simulink model "HPWnew"  (R2015a)
settings: Solver=ode45  StartTime=0.0  StopTime=10.0  RelTol=1e-3
undefined symbols (not defined in the file): c1, c2, c3, c4, c5, c6, Hydride, Metal, Nickel, PV1, PV2, PV3
libraries: powerlib x263, electricdrivelib x30, powerlib_meascontrol x15, powerlib_extras x7, re_lib x3, fuzblock x3, simulink x2
(part 4 of 8)

== system HPWnew/Wind Power System 60 KW x 25 = 1.5MW/Wind 60KW, 50HZ, 440V19 ==
  "Gen Speed " : Inport
  PA (deg) : Inport  Port=2
  Wind Speed (m/s) : Inport  Port=3
  Ground (output) : powerlib/Elements/Ground  LConnTagsString=a
  Load Flow Bus : powerlib/Measurements/Load Flow Bus  LConnTagsString=a  ID=B1  Vbase=762.1  Vref=1  Vangle=0  VLF=1  angleLF=-0.3472
      settings: AttributesFormatString=%<ID>\n%<Vbase>V\n%<VLF>pu\n%<angleLF>deg.
  Network 440Vrms LN - 10 MVA : powerlib/Electrical Sources/Three-Phase Source  Voltage=(762.1)*1  PhaseAngle=0  Frequency=60  InternalConnection=Yn  SpecifyImpedance=off  Resistance=762^2/10e6/10  Inductance=762^2/10e6/(2*pi*60)  ShortCircuitLevel=100e6  BaseVoltage=25e3  XRratio=7  BusType=swing  Pref=0  Qref=0  Qmin=-Inf  Qmax=Inf
  Scope : Scope  NumInputPorts=2
      settings: TimeRange=0.05586047612700701  YMin=-800~-200  YMax=800~200
  Synchronous Machine 762 V 111.9 kW : powerlib/Machines/Synchronous Machine SI Fundamental  PresetModel=05: 50Hz 400V 60kVA 1500RPM  MechanicalLoad=Mechanical power Pm  ShowDetailedParameters=on  RotorType=Salient-pole  Units=SI fundamental parameters  MeasurementBus=off  NominalParameters=[6e+04 400 50]  Stator=[0.101 0.0006791 0.01833 0.007979]  Field=[0.05664 0.001459]  Dampers2=[ 1 2 3 4 5 6 ]  Dampers1=[0.3901 0.002619 0.1534 0.0004483]  Mechanical=[0.5 0.05 2]  PolePairs=2  InitialConditions=[0 -111.483 53.977 53.977 53.977 -173.297 -293.297 -53.2967 17.8876]  SetSaturation=off  Saturation=[46.376,51.647,61.167,66.773,72.147,78.393,86.24,95.347,105.58;644,708.2,816.2,870.87,917.13,962.47,1012,1059.3,1104.5]  DisplayVfd=off  LoadFlowParameters=[1 -50000 0 0 0]  TsPowergui=0  TsBlock=-1  IterativeModel=Forward Euler  BusType=PV  Pref=-50000  Qref=0  Qmin=-Inf  Qmax=Inf  PLF=0  QLF=0
      settings: AttributesFormatString=\n
  Three-Phase Series RLC Load : powerlib/Elements/Three-Phase Series RLC Load  LConnTagsString=A|B|C  Configuration=Y (grounded)  NominalVoltage=440  NominalFrequency=50  ActivePower=10e3  InductivePower=0  CapacitivePower=0  Measurements=None  LoadType=constant Z
  Three-Phase V-I Measurement : powerlib/Measurements/Three-Phase V-I Measurement  VoltageMeasurement=phase-to-ground  SetLabelV=off  LabelV=Vabc  Vpu=off  VpuLL=off  CurrentMeasurement=yes  SetLabelI=off  LabelI=Iabc  Ipu=off  Pbase=100e6  Vbase=500e3  OutputType=Complex  PhasorSimulation=off  PSBequivalent=0
  Wind Turbine : Subsystem  AncestorBlock=re_lib/Wind Generation/Wind Turbine  DialogController=POWERSYS.PowerSysDialog  mask(Wind Turbine){Pnom=1.5e6, Pelec_base=1.5e6/0.9, wind_base=12, P_wind_base=0.73, speed_nom=1.2, pitch_angle=0, DisplayTurbChar=off, c1_c6=[0.51763          116          0.4            5           21     0.006795], cp_nom=0.48, lambda_nom=8.1}
      mask prompts: Pnom "Nominal mechanical output power (W):"; Pelec_base "Base power of the electrical generator (VA):"; wind_base "Base wind speed (m/s):"; P_wind_base "Maximum power at base wind speed (pu of nominal mechanical power):"; speed_nom "Base rotational speed (p.u. of base generator speed):"; pitch_angle "Pitch angle beta to display wind-turbine power characteristics (beta >=0)  (deg):"; DisplayTurbChar "Display wind turbine power characteristics"
      mask help:
      | This block implements a variable pitch wind turbine model. The performance coefficient Cp of the turbine is the mechanical output power of the turbine divided by wind power and a function of wind speed, rotational speed, and pitch angle (beta). Cp reaches its maximum value at zero beta. Select the wind-turbine power characteristics display to plot the turbine characteristics at the specified pitch angle.
      |
      | The first input is the generator speed in per unit of the generator base speed. For a synchronous or asynchronous generator, the base speed is the synchronous speed. For a permanent-magnet generator, the base speed is defined as the speed producing nominal voltage at  no load. The second input is the blade pitch angle (beta) in degrees. The third input is the wind speed in m/s.
      |
      | The output is the torque applied to the generator shaft in per unit of the generator ratings.
      |
      | The turbine inertia must be added to the generator inertia.
      mask init: same as HPWnew/Wind Power System 60 KW x 25 = 1.5MW/Wind 60KW, 50HZ, 440V1/Wind Turbine
      mask Help: helpview(psbhelp);
      mask Callback Pnom:
      | ParVisible={'on','on','on','on','on','on','on','off','off','off',};
      | set_param(gcb,'MaskVisibilities',ParVisible);
      | c1_c6=str2num(get_param(gcb,'c1_c6'));
      | c1=c1_c6(1);c2=c1_c6(2);c3=c1_c6(3);c4=c1_c6(4);c5=c1_c6(5);c6=c1_c6(6);
      mask Callback DisplayTurbChar:
      | DisplayTurbChar=get_param(gcb,'DisplayTurbChar');
      | 
      | if strcmp(DisplayTurbChar,'on')
      |     fig_num=figure;
      | 	clf(fig_num);
      | 	[speed_nom,wind_base,P_wind_base,pitch_angle]=getSPSmaskvalues(gcb,{'speed_nom','wind_base','P_wind_base','pitch_angle'});
      | 	[c1_c6,lambda_nom,cp_nom]=getSPSmaskvalues(gcb,{'c1_c6','lambda_nom','cp_nom'});
      | 	c1=c1_c6(1);c2=c1_c6(2);c3=c1_c6(3);c4=c1_c6(4);c5=c1_c6(5);c6=c1_c6(6);
      | 
      | 	%Wind turbine typical characteristic data
      |     %c2=116;c3=0.4;c4=5;c5=21;
      |     %Computation of c1 and c6 for lambda_nom et cpmax
      |     %lambda_nom=8.1;
      |     %cp_max=0.48;
      |     %cp_nom=cp_max;
      | 
      |     %lambda_i_nom=1/(1/lambda_nom-0.035);
      |     %k_nom=-(c2*c5/lambda_i_nom-c4*c5-c2)*exp(-c5/lambda_i_nom)/lambda_nom^2;
      |     %c1=cp_max/((c2/lambda_i_nom-c4)*exp(-c5/lambda_i_nom)+k_nom*lambda_nom);
      |     %c6=k_nom*c1;
      | 
      | 	wr_elec_pu=1e-3:0.01:1.5;;
      |     wr_mec_pu=wr_elec_pu/speed_nom;
      |     wind_max=ceil((1.2/P_wind_base)^(1/3)*wind_base);
      |     wind_min=round(((0.1)/P_wind_base)^(1/3)*wind_base);
      |     wind1=wind_min:(wind_base-wind_min)/5:wind_base;
      |     wind2=wind_base+(wind_base-wind_min)/5:(wind_base-wind_min)/5:wind_max;
      |     wind_pu=[wind1 wind2]/wind_base;
      | 
      |     for k=1:length(wind_pu)
      |         for i=1:length(wr_mec_pu);
      |             lambda_pu=wr_mec_pu(i)/wind_pu(k);
      |             lambda=lambda_pu*lambda_nom;
      |             lambda_i=1/(1/(lambda+0.08*pitch_angle)-0.035/(pitch_angle^3+1));
      |             cp=c1*(c2/lambda_i-c3*pitch_angle-c4)*exp(-c5/lambda_i)+c6*lambda;
      |             cp_pu=cp/cp_nom;
      |             Pwind_pu(k,i)=wind_pu(k)^3*cp_pu*P_wind_base;
      |         end
      |     end
      |     for k=1:length(wind_pu)
      |         plot(wr_elec_pu,Pwind_pu(k,:))
      |         hold on
      |     end
      | 
      |     plot([speed_nom,speed_nom,0],[0,P_wind_base,P_wind_base],'r--')
      |     text(speed_nom+0.01,0+0.05,sprintf('%0.4g pu',speed_nom))
      |     text(0.01,P_wind_base+0.05,sprintf('Max. power at base wind speed (%0.4g m/s) and beta = 0 deg',wind_base))
      |     for i=1:length(wind_pu),
      |         p_max(i)=max(Pwind_pu(i,:));
      |         speed(i)=wr_elec_pu(find(Pwind_pu(i,:)==p_max(i)));
      |         text(speed(i),p_max(i),sprintf('%0.4g m/s',wind_pu(i)*wind_base))
      |     end
      |     plot([0 max(wr_elec_pu)],[0 0],'--')
      | 
      |     xlabel('Turbine speed (pu of nominal generator speed)')
      |     ylabel('Turbine output power (pu of nominal mechanical power)')
      |     title(sprintf('Turbine Power Characteristics (Pitch angle beta = %0.4g deg)',pitch_angle))
      |     axis([0 max(wr_elec_pu) min(Pwind_pu(1,:)) max(P_wind_base+0.1,max(wind_pu)^3*P_wind_base+0.1)])
      |     set_param(gcb,'DisplayTurbChar','off')
      | end
      mask Display: disp('');
  i mach : powerlib/Measurements/Current Measurement  Tag=PoWeRsYsTeMmEaSuReMeNt  PhasorSimulation=off  OutputType=Magnitude  PSBequivalent=0
  iA (A) : Scope
      settings: TickLabels=on  TimeRange=3  YMin=-100  YMax=100  SaveName=is1
  vf : Constant  Value=17.888
  A : PMIOPort  Port=1  Side=Right
  B : PMIOPort  Port=2  Side=Right
  C : PMIOPort  Port=3  Side=Right
  wires:
  Three-Phase V-I Measurement/2 -> Scope/2
  Three-Phase V-I Measurement/1 -> Scope/1
  PA (deg)/1 -> Wind Turbine/2(Pitch angle (deg))
  Wind Speed (m/s)/1 -> Wind Turbine/3(Wind speed (m/s))
  "Gen Speed "/1 -> Wind Turbine/1(Generator speed (pu))
  Wind Turbine/1("Tm ") -> Synchronous Machine 762 V 111.9 kW/1
  vf/1 -> Synchronous Machine 762 V 111.9 kW/2
  i mach/1 -> iA (A)/1
  connections:
  Three-Phase V-I Measurement/LConn3 -- Synchronous Machine 762 V 111.9 kW/RConn3
  Three-Phase V-I Measurement/LConn1 -- Synchronous Machine 762 V 111.9 kW/RConn1
  Three-Phase V-I Measurement/LConn2 -- Synchronous Machine 762 V 111.9 kW/RConn2
  Three-Phase V-I Measurement/RConn1 -- i mach/LConn1
  Ground (output)/LConn1 -- Network 440Vrms LN - 10 MVA/LConn1
  i mach/RConn1 -- Three-Phase Series RLC Load/LConn1 -- Load Flow Bus/LConn1 -- Network 440Vrms LN - 10 MVA/RConn1 -- A/RConn1
  Three-Phase Series RLC Load/LConn3 -- Three-Phase V-I Measurement/RConn3 -- Network 440Vrms LN - 10 MVA/RConn3 -- C/RConn1
  Network 440Vrms LN - 10 MVA/RConn2 -- Three-Phase V-I Measurement/RConn2 -- Three-Phase Series RLC Load/LConn2 -- B/RConn1

== system HPWnew/Wind Power System 60 KW x 25 = 1.5MW/Wind 60KW, 50HZ, 440V2 ==
  "Gen Speed " : Inport
  PA (deg) : Inport  Port=2
  Wind Speed (m/s) : Inport  Port=3
  Ground (output) : powerlib/Elements/Ground  LConnTagsString=a
  Load Flow Bus : powerlib/Measurements/Load Flow Bus  LConnTagsString=a  ID=B1  Vbase=762.1  Vref=1  Vangle=0  VLF=1  angleLF=-0.3472
      settings: AttributesFormatString=%<ID>\n%<Vbase>V\n%<VLF>pu\n%<angleLF>deg.
  Network 440Vrms LN - 10 MVA : powerlib/Electrical Sources/Three-Phase Source  Voltage=(762.1)*1  PhaseAngle=0  Frequency=60  InternalConnection=Yn  SpecifyImpedance=off  Resistance=762^2/10e6/10  Inductance=762^2/10e6/(2*pi*60)  ShortCircuitLevel=100e6  BaseVoltage=25e3  XRratio=7  BusType=swing  Pref=0  Qref=0  Qmin=-Inf  Qmax=Inf
  Scope : Scope  NumInputPorts=2
      settings: TimeRange=0.05586047612700701  YMin=-800~-200  YMax=800~200
  Synchronous Machine 762 V 111.9 kW : powerlib/Machines/Synchronous Machine SI Fundamental  PresetModel=05: 50Hz 400V 60kVA 1500RPM  MechanicalLoad=Mechanical power Pm  ShowDetailedParameters=on  RotorType=Salient-pole  Units=SI fundamental parameters  MeasurementBus=off  NominalParameters=[6e+04 400 50]  Stator=[0.101 0.0006791 0.01833 0.007979]  Field=[0.05664 0.001459]  Dampers2=[ 1 2 3 4 5 6 ]  Dampers1=[0.3901 0.002619 0.1534 0.0004483]  Mechanical=[0.5 0.05 2]  PolePairs=2  InitialConditions=[0 -111.483 53.977 53.977 53.977 -173.297 -293.297 -53.2967 17.8876]  SetSaturation=off  Saturation=[46.376,51.647,61.167,66.773,72.147,78.393,86.24,95.347,105.58;644,708.2,816.2,870.87,917.13,962.47,1012,1059.3,1104.5]  DisplayVfd=off  LoadFlowParameters=[1 -50000 0 0 0]  TsPowergui=0  TsBlock=-1  IterativeModel=Forward Euler  BusType=PV  Pref=-50000  Qref=0  Qmin=-Inf  Qmax=Inf  PLF=0  QLF=0
      settings: AttributesFormatString=\n
  Three-Phase Series RLC Load : powerlib/Elements/Three-Phase Series RLC Load  LConnTagsString=A|B|C  Configuration=Y (grounded)  NominalVoltage=440  NominalFrequency=50  ActivePower=10e3  InductivePower=0  CapacitivePower=0  Measurements=None  LoadType=constant Z
  Three-Phase V-I Measurement : powerlib/Measurements/Three-Phase V-I Measurement  VoltageMeasurement=phase-to-ground  SetLabelV=off  LabelV=Vabc  Vpu=off  VpuLL=off  CurrentMeasurement=yes  SetLabelI=off  LabelI=Iabc  Ipu=off  Pbase=100e6  Vbase=500e3  OutputType=Complex  PhasorSimulation=off  PSBequivalent=0
  Wind Turbine : Subsystem  AncestorBlock=re_lib/Wind Generation/Wind Turbine  DialogController=POWERSYS.PowerSysDialog  mask(Wind Turbine){Pnom=1.5e6, Pelec_base=1.5e6/0.9, wind_base=12, P_wind_base=0.73, speed_nom=1.2, pitch_angle=0, DisplayTurbChar=off, c1_c6=[0.51763          116          0.4            5           21     0.006795], cp_nom=0.48, lambda_nom=8.1}
      mask prompts: Pnom "Nominal mechanical output power (W):"; Pelec_base "Base power of the electrical generator (VA):"; wind_base "Base wind speed (m/s):"; P_wind_base "Maximum power at base wind speed (pu of nominal mechanical power):"; speed_nom "Base rotational speed (p.u. of base generator speed):"; pitch_angle "Pitch angle beta to display wind-turbine power characteristics (beta >=0)  (deg):"; DisplayTurbChar "Display wind turbine power characteristics"
      mask help:
      | This block implements a variable pitch wind turbine model. The performance coefficient Cp of the turbine is the mechanical output power of the turbine divided by wind power and a function of wind speed, rotational speed, and pitch angle (beta). Cp reaches its maximum value at zero beta. Select the wind-turbine power characteristics display to plot the turbine characteristics at the specified pitch angle.
      |
      | The first input is the generator speed in per unit of the generator base speed. For a synchronous or asynchronous generator, the base speed is the synchronous speed. For a permanent-magnet generator, the base speed is defined as the speed producing nominal voltage at  no load. The second input is the blade pitch angle (beta) in degrees. The third input is the wind speed in m/s.
      |
      | The output is the torque applied to the generator shaft in per unit of the generator ratings.
      |
      | The turbine inertia must be added to the generator inertia.
      mask init: same as HPWnew/Wind Power System 60 KW x 25 = 1.5MW/Wind 60KW, 50HZ, 440V1/Wind Turbine
      mask Help: helpview(psbhelp);
      mask Callback Pnom:
      | ParVisible={'on','on','on','on','on','on','on','off','off','off',};
      | set_param(gcb,'MaskVisibilities',ParVisible);
      | c1_c6=str2num(get_param(gcb,'c1_c6'));
      | c1=c1_c6(1);c2=c1_c6(2);c3=c1_c6(3);c4=c1_c6(4);c5=c1_c6(5);c6=c1_c6(6);
      mask Callback DisplayTurbChar:
      | DisplayTurbChar=get_param(gcb,'DisplayTurbChar');
      | 
      | if strcmp(DisplayTurbChar,'on')
      |     fig_num=figure;
      | 	clf(fig_num);
      | 	[speed_nom,wind_base,P_wind_base,pitch_angle]=getSPSmaskvalues(gcb,{'speed_nom','wind_base','P_wind_base','pitch_angle'});
      | 	[c1_c6,lambda_nom,cp_nom]=getSPSmaskvalues(gcb,{'c1_c6','lambda_nom','cp_nom'});
      | 	c1=c1_c6(1);c2=c1_c6(2);c3=c1_c6(3);c4=c1_c6(4);c5=c1_c6(5);c6=c1_c6(6);
      | 
      | 	%Wind turbine typical characteristic data
      |     %c2=116;c3=0.4;c4=5;c5=21;
      |     %Computation of c1 and c6 for lambda_nom et cpmax
      |     %lambda_nom=8.1;
      |     %cp_max=0.48;
      |     %cp_nom=cp_max;
      | 
      |     %lambda_i_nom=1/(1/lambda_nom-0.035);
      |     %k_nom=-(c2*c5/lambda_i_nom-c4*c5-c2)*exp(-c5/lambda_i_nom)/lambda_nom^2;
      |     %c1=cp_max/((c2/lambda_i_nom-c4)*exp(-c5/lambda_i_nom)+k_nom*lambda_nom);
      |     %c6=k_nom*c1;
      | 
      | 	wr_elec_pu=1e-3:0.01:1.5;;
      |     wr_mec_pu=wr_elec_pu/speed_nom;
      |     wind_max=ceil((1.2/P_wind_base)^(1/3)*wind_base);
      |     wind_min=round(((0.1)/P_wind_base)^(1/3)*wind_base);
      |     wind1=wind_min:(wind_base-wind_min)/5:wind_base;
      |     wind2=wind_base+(wind_base-wind_min)/5:(wind_base-wind_min)/5:wind_max;
      |     wind_pu=[wind1 wind2]/wind_base;
      | 
      |     for k=1:length(wind_pu)
      |         for i=1:length(wr_mec_pu);
      |             lambda_pu=wr_mec_pu(i)/wind_pu(k);
      |             lambda=lambda_pu*lambda_nom;
      |             lambda_i=1/(1/(lambda+0.08*pitch_angle)-0.035/(pitch_angle^3+1));
      |             cp=c1*(c2/lambda_i-c3*pitch_angle-c4)*exp(-c5/lambda_i)+c6*lambda;
      |             cp_pu=cp/cp_nom;
      |             Pwind_pu(k,i)=wind_pu(k)^3*cp_pu*P_wind_base;
      |         end
      |     end
      |     for k=1:length(wind_pu)
      |         plot(wr_elec_pu,Pwind_pu(k,:))
      |         hold on
      |     end
      | 
      |     plot([speed_nom,speed_nom,0],[0,P_wind_base,P_wind_base],'r--')
      |     text(speed_nom+0.01,0+0.05,sprintf('%0.4g pu',speed_nom))
      |     text(0.01,P_wind_base+0.05,sprintf('Max. power at base wind speed (%0.4g m/s) and beta = 0 deg',wind_base))
      |     for i=1:length(wind_pu),
      |         p_max(i)=max(Pwind_pu(i,:));
      |         speed(i)=wr_elec_pu(find(Pwind_pu(i,:)==p_max(i)));
      |         text(speed(i),p_max(i),sprintf('%0.4g m/s',wind_pu(i)*wind_base))
      |     end
      |     plot([0 max(wr_elec_pu)],[0 0],'--')
      | 
      |     xlabel('Turbine speed (pu of nominal generator speed)')
      |     ylabel('Turbine output power (pu of nominal mechanical power)')
      |     title(sprintf('Turbine Power Characteristics (Pitch angle beta = %0.4g deg)',pitch_angle))
      |     axis([0 max(wr_elec_pu) min(Pwind_pu(1,:)) max(P_wind_base+0.1,max(wind_pu)^3*P_wind_base+0.1)])
      |     set_param(gcb,'DisplayTurbChar','off')
      | end
      mask Display: disp('');
  i mach : powerlib/Measurements/Current Measurement  Tag=PoWeRsYsTeMmEaSuReMeNt  PhasorSimulation=off  OutputType=Magnitude  PSBequivalent=0
  iA (A) : Scope
      settings: TickLabels=on  TimeRange=3  YMin=-100  YMax=100  SaveName=is1
  vf : Constant  Value=17.888
  A : PMIOPort  Port=1  Side=Right
  B : PMIOPort  Port=2  Side=Right
  C : PMIOPort  Port=3  Side=Right
  wires:
  Three-Phase V-I Measurement/2 -> Scope/2
  Three-Phase V-I Measurement/1 -> Scope/1
  PA (deg)/1 -> Wind Turbine/2(Pitch angle (deg))
  Wind Speed (m/s)/1 -> Wind Turbine/3(Wind speed (m/s))
  "Gen Speed "/1 -> Wind Turbine/1(Generator speed (pu))
  Wind Turbine/1("Tm ") -> Synchronous Machine 762 V 111.9 kW/1
  vf/1 -> Synchronous Machine 762 V 111.9 kW/2
  i mach/1 -> iA (A)/1
  connections:
  Three-Phase V-I Measurement/LConn3 -- Synchronous Machine 762 V 111.9 kW/RConn3
  Three-Phase V-I Measurement/LConn1 -- Synchronous Machine 762 V 111.9 kW/RConn1
  Three-Phase V-I Measurement/LConn2 -- Synchronous Machine 762 V 111.9 kW/RConn2
  Three-Phase V-I Measurement/RConn1 -- i mach/LConn1
  Ground (output)/LConn1 -- Network 440Vrms LN - 10 MVA/LConn1
  i mach/RConn1 -- Three-Phase Series RLC Load/LConn1 -- Load Flow Bus/LConn1 -- Network 440Vrms LN - 10 MVA/RConn1 -- A/RConn1
  Three-Phase Series RLC Load/LConn3 -- Three-Phase V-I Measurement/RConn3 -- Network 440Vrms LN - 10 MVA/RConn3 -- C/RConn1
  Network 440Vrms LN - 10 MVA/RConn2 -- Three-Phase V-I Measurement/RConn2 -- Three-Phase Series RLC Load/LConn2 -- B/RConn1

== system HPWnew/Wind Power System 60 KW x 25 = 1.5MW/Wind 60KW, 50HZ, 440V20 ==
  "Gen Speed " : Inport
  PA (deg) : Inport  Port=2
  Wind Speed (m/s) : Inport  Port=3
  Ground (output) : powerlib/Elements/Ground  LConnTagsString=a
  Load Flow Bus : powerlib/Measurements/Load Flow Bus  LConnTagsString=a  ID=B1  Vbase=762.1  Vref=1  Vangle=0  VLF=1  angleLF=-0.3472
      settings: AttributesFormatString=%<ID>\n%<Vbase>V\n%<VLF>pu\n%<angleLF>deg.
  Network 440Vrms LN - 10 MVA : powerlib/Electrical Sources/Three-Phase Source  Voltage=(762.1)*1  PhaseAngle=0  Frequency=60  InternalConnection=Yn  SpecifyImpedance=off  Resistance=762^2/10e6/10  Inductance=762^2/10e6/(2*pi*60)  ShortCircuitLevel=100e6  BaseVoltage=25e3  XRratio=7  BusType=swing  Pref=0  Qref=0  Qmin=-Inf  Qmax=Inf
  Scope : Scope  NumInputPorts=2
      settings: TimeRange=0.05586047612700701  YMin=-800~-200  YMax=800~200
  Synchronous Machine 762 V 111.9 kW : powerlib/Machines/Synchronous Machine SI Fundamental  PresetModel=05: 50Hz 400V 60kVA 1500RPM  MechanicalLoad=Mechanical power Pm  ShowDetailedParameters=on  RotorType=Salient-pole  Units=SI fundamental parameters  MeasurementBus=off  NominalParameters=[6e+04 400 50]  Stator=[0.101 0.0006791 0.01833 0.007979]  Field=[0.05664 0.001459]  Dampers2=[ 1 2 3 4 5 6 ]  Dampers1=[0.3901 0.002619 0.1534 0.0004483]  Mechanical=[0.5 0.05 2]  PolePairs=2  InitialConditions=[0 -111.483 53.977 53.977 53.977 -173.297 -293.297 -53.2967 17.8876]  SetSaturation=off  Saturation=[46.376,51.647,61.167,66.773,72.147,78.393,86.24,95.347,105.58;644,708.2,816.2,870.87,917.13,962.47,1012,1059.3,1104.5]  DisplayVfd=off  LoadFlowParameters=[1 -50000 0 0 0]  TsPowergui=0  TsBlock=-1  IterativeModel=Forward Euler  BusType=PV  Pref=-50000  Qref=0  Qmin=-Inf  Qmax=Inf  PLF=0  QLF=0
      settings: AttributesFormatString=\n
  Three-Phase Series RLC Load : powerlib/Elements/Three-Phase Series RLC Load  LConnTagsString=A|B|C  Configuration=Y (grounded)  NominalVoltage=440  NominalFrequency=50  ActivePower=10e3  InductivePower=0  CapacitivePower=0  Measurements=None  LoadType=constant Z
  Three-Phase V-I Measurement : powerlib/Measurements/Three-Phase V-I Measurement  VoltageMeasurement=phase-to-ground  SetLabelV=off  LabelV=Vabc  Vpu=off  VpuLL=off  CurrentMeasurement=yes  SetLabelI=off  LabelI=Iabc  Ipu=off  Pbase=100e6  Vbase=500e3  OutputType=Complex  PhasorSimulation=off  PSBequivalent=0
  Wind Turbine : Subsystem  AncestorBlock=re_lib/Wind Generation/Wind Turbine  DialogController=POWERSYS.PowerSysDialog  mask(Wind Turbine){Pnom=1.5e6, Pelec_base=1.5e6/0.9, wind_base=12, P_wind_base=0.73, speed_nom=1.2, pitch_angle=0, DisplayTurbChar=off, c1_c6=[0.51763          116          0.4            5           21     0.006795], cp_nom=0.48, lambda_nom=8.1}
      mask prompts: Pnom "Nominal mechanical output power (W):"; Pelec_base "Base power of the electrical generator (VA):"; wind_base "Base wind speed (m/s):"; P_wind_base "Maximum power at base wind speed (pu of nominal mechanical power):"; speed_nom "Base rotational speed (p.u. of base generator speed):"; pitch_angle "Pitch angle beta to display wind-turbine power characteristics (beta >=0)  (deg):"; DisplayTurbChar "Display wind turbine power characteristics"
      mask help:
      | This block implements a variable pitch wind turbine model. The performance coefficient Cp of the turbine is the mechanical output power of the turbine divided by wind power and a function of wind speed, rotational speed, and pitch angle (beta). Cp reaches its maximum value at zero beta. Select the wind-turbine power characteristics display to plot the turbine characteristics at the specified pitch angle.
      |
      | The first input is the generator speed in per unit of the generator base speed. For a synchronous or asynchronous generator, the base speed is the synchronous speed. For a permanent-magnet generator, the base speed is defined as the speed producing nominal voltage at  no load. The second input is the blade pitch angle (beta) in degrees. The third input is the wind speed in m/s.
      |
      | The output is the torque applied to the generator shaft in per unit of the generator ratings.
      |
      | The turbine inertia must be added to the generator inertia.
      mask init: same as HPWnew/Wind Power System 60 KW x 25 = 1.5MW/Wind 60KW, 50HZ, 440V1/Wind Turbine
      mask Help: helpview(psbhelp);
      mask Callback Pnom:
      | ParVisible={'on','on','on','on','on','on','on','off','off','off',};
      | set_param(gcb,'MaskVisibilities',ParVisible);
      | c1_c6=str2num(get_param(gcb,'c1_c6'));
      | c1=c1_c6(1);c2=c1_c6(2);c3=c1_c6(3);c4=c1_c6(4);c5=c1_c6(5);c6=c1_c6(6);
      mask Callback DisplayTurbChar:
      | DisplayTurbChar=get_param(gcb,'DisplayTurbChar');
      | 
      | if strcmp(DisplayTurbChar,'on')
      |     fig_num=figure;
      | 	clf(fig_num);
      | 	[speed_nom,wind_base,P_wind_base,pitch_angle]=getSPSmaskvalues(gcb,{'speed_nom','wind_base','P_wind_base','pitch_angle'});
      | 	[c1_c6,lambda_nom,cp_nom]=getSPSmaskvalues(gcb,{'c1_c6','lambda_nom','cp_nom'});
      | 	c1=c1_c6(1);c2=c1_c6(2);c3=c1_c6(3);c4=c1_c6(4);c5=c1_c6(5);c6=c1_c6(6);
      | 
      | 	%Wind turbine typical characteristic data
      |     %c2=116;c3=0.4;c4=5;c5=21;
      |     %Computation of c1 and c6 for lambda_nom et cpmax
      |     %lambda_nom=8.1;
      |     %cp_max=0.48;
      |     %cp_nom=cp_max;
      | 
      |     %lambda_i_nom=1/(1/lambda_nom-0.035);
      |     %k_nom=-(c2*c5/lambda_i_nom-c4*c5-c2)*exp(-c5/lambda_i_nom)/lambda_nom^2;
      |     %c1=cp_max/((c2/lambda_i_nom-c4)*exp(-c5/lambda_i_nom)+k_nom*lambda_nom);
      |     %c6=k_nom*c1;
      | 
      | 	wr_elec_pu=1e-3:0.01:1.5;;
      |     wr_mec_pu=wr_elec_pu/speed_nom;
      |     wind_max=ceil((1.2/P_wind_base)^(1/3)*wind_base);
      |     wind_min=round(((0.1)/P_wind_base)^(1/3)*wind_base);
      |     wind1=wind_min:(wind_base-wind_min)/5:wind_base;
      |     wind2=wind_base+(wind_base-wind_min)/5:(wind_base-wind_min)/5:wind_max;
      |     wind_pu=[wind1 wind2]/wind_base;
      | 
      |     for k=1:length(wind_pu)
      |         for i=1:length(wr_mec_pu);
      |             lambda_pu=wr_mec_pu(i)/wind_pu(k);
      |             lambda=lambda_pu*lambda_nom;
      |             lambda_i=1/(1/(lambda+0.08*pitch_angle)-0.035/(pitch_angle^3+1));
      |             cp=c1*(c2/lambda_i-c3*pitch_angle-c4)*exp(-c5/lambda_i)+c6*lambda;
      |             cp_pu=cp/cp_nom;
      |             Pwind_pu(k,i)=wind_pu(k)^3*cp_pu*P_wind_base;
      |         end
      |     end
      |     for k=1:length(wind_pu)
      |         plot(wr_elec_pu,Pwind_pu(k,:))
      |         hold on
      |     end
      | 
      |     plot([speed_nom,speed_nom,0],[0,P_wind_base,P_wind_base],'r--')
      |     text(speed_nom+0.01,0+0.05,sprintf('%0.4g pu',speed_nom))
      |     text(0.01,P_wind_base+0.05,sprintf('Max. power at base wind speed (%0.4g m/s) and beta = 0 deg',wind_base))
      |     for i=1:length(wind_pu),
      |         p_max(i)=max(Pwind_pu(i,:));
      |         speed(i)=wr_elec_pu(find(Pwind_pu(i,:)==p_max(i)));
      |         text(speed(i),p_max(i),sprintf('%0.4g m/s',wind_pu(i)*wind_base))
      |     end
      |     plot([0 max(wr_elec_pu)],[0 0],'--')
      | 
      |     xlabel('Turbine speed (pu of nominal generator speed)')
      |     ylabel('Turbine output power (pu of nominal mechanical power)')
      |     title(sprintf('Turbine Power Characteristics (Pitch angle beta = %0.4g deg)',pitch_angle))
      |     axis([0 max(wr_elec_pu) min(Pwind_pu(1,:)) max(P_wind_base+0.1,max(wind_pu)^3*P_wind_base+0.1)])
      |     set_param(gcb,'DisplayTurbChar','off')
      | end
      mask Display: disp('');
  i mach : powerlib/Measurements/Current Measurement  Tag=PoWeRsYsTeMmEaSuReMeNt  PhasorSimulation=off  OutputType=Magnitude  PSBequivalent=0
  iA (A) : Scope
      settings: TickLabels=on  TimeRange=3  YMin=-100  YMax=100  SaveName=is1
  vf : Constant  Value=17.888
  A : PMIOPort  Port=1  Side=Right
  B : PMIOPort  Port=2  Side=Right
  C : PMIOPort  Port=3  Side=Right
  wires:
  i mach/1 -> iA (A)/1
  vf/1 -> Synchronous Machine 762 V 111.9 kW/2
  Wind Turbine/1("Tm ") -> Synchronous Machine 762 V 111.9 kW/1
  "Gen Speed "/1 -> Wind Turbine/1(Generator speed (pu))
  Wind Speed (m/s)/1 -> Wind Turbine/3(Wind speed (m/s))
  PA (deg)/1 -> Wind Turbine/2(Pitch angle (deg))
  Three-Phase V-I Measurement/1 -> Scope/1
  Three-Phase V-I Measurement/2 -> Scope/2
  connections:
  B/RConn1 -- Three-Phase Series RLC Load/LConn2 -- Three-Phase V-I Measurement/RConn2 -- Network 440Vrms LN - 10 MVA/RConn2
  C/RConn1 -- Network 440Vrms LN - 10 MVA/RConn3 -- Three-Phase V-I Measurement/RConn3 -- Three-Phase Series RLC Load/LConn3
  A/RConn1 -- Network 440Vrms LN - 10 MVA/RConn1 -- Load Flow Bus/LConn1 -- Three-Phase Series RLC Load/LConn1 -- i mach/RConn1
  Ground (output)/LConn1 -- Network 440Vrms LN - 10 MVA/LConn1
  Three-Phase V-I Measurement/RConn1 -- i mach/LConn1
  Three-Phase V-I Measurement/LConn2 -- Synchronous Machine 762 V 111.9 kW/RConn2
  Three-Phase V-I Measurement/LConn1 -- Synchronous Machine 762 V 111.9 kW/RConn1
  Three-Phase V-I Measurement/LConn3 -- Synchronous Machine 762 V 111.9 kW/RConn3

== system HPWnew/Wind Power System 60 KW x 25 = 1.5MW/Wind 60KW, 50HZ, 440V21 ==
  "Gen Speed " : Inport
  PA (deg) : Inport  Port=2
  Wind Speed (m/s) : Inport  Port=3
  Ground (output) : powerlib/Elements/Ground  LConnTagsString=a
  Load Flow Bus : powerlib/Measurements/Load Flow Bus  LConnTagsString=a  ID=B1  Vbase=762.1  Vref=1  Vangle=0  VLF=1  angleLF=-0.3472
      settings: AttributesFormatString=%<ID>\n%<Vbase>V\n%<VLF>pu\n%<angleLF>deg.
  Network 440Vrms LN - 10 MVA : powerlib/Electrical Sources/Three-Phase Source  Voltage=(762.1)*1  PhaseAngle=0  Frequency=60  InternalConnection=Yn  SpecifyImpedance=off  Resistance=762^2/10e6/10  Inductance=762^2/10e6/(2*pi*60)  ShortCircuitLevel=100e6  BaseVoltage=25e3  XRratio=7  BusType=swing  Pref=0  Qref=0  Qmin=-Inf  Qmax=Inf
  Scope : Scope  NumInputPorts=2
      settings: TimeRange=0.05586047612700701  YMin=-800~-200  YMax=800~200
  Synchronous Machine 762 V 111.9 kW : powerlib/Machines/Synchronous Machine SI Fundamental  PresetModel=05: 50Hz 400V 60kVA 1500RPM  MechanicalLoad=Mechanical power Pm  ShowDetailedParameters=on  RotorType=Salient-pole  Units=SI fundamental parameters  MeasurementBus=off  NominalParameters=[6e+04 400 50]  Stator=[0.101 0.0006791 0.01833 0.007979]  Field=[0.05664 0.001459]  Dampers2=[ 1 2 3 4 5 6 ]  Dampers1=[0.3901 0.002619 0.1534 0.0004483]  Mechanical=[0.5 0.05 2]  PolePairs=2  InitialConditions=[0 -111.483 53.977 53.977 53.977 -173.297 -293.297 -53.2967 17.8876]  SetSaturation=off  Saturation=[46.376,51.647,61.167,66.773,72.147,78.393,86.24,95.347,105.58;644,708.2,816.2,870.87,917.13,962.47,1012,1059.3,1104.5]  DisplayVfd=off  LoadFlowParameters=[1 -50000 0 0 0]  TsPowergui=0  TsBlock=-1  IterativeModel=Forward Euler  BusType=PV  Pref=-50000  Qref=0  Qmin=-Inf  Qmax=Inf  PLF=0  QLF=0
      settings: AttributesFormatString=\n
  Three-Phase Series RLC Load : powerlib/Elements/Three-Phase Series RLC Load  LConnTagsString=A|B|C  Configuration=Y (grounded)  NominalVoltage=440  NominalFrequency=50  ActivePower=10e3  InductivePower=0  CapacitivePower=0  Measurements=None  LoadType=constant Z
  Three-Phase V-I Measurement : powerlib/Measurements/Three-Phase V-I Measurement  VoltageMeasurement=phase-to-ground  SetLabelV=off  LabelV=Vabc  Vpu=off  VpuLL=off  CurrentMeasurement=yes  SetLabelI=off  LabelI=Iabc  Ipu=off  Pbase=100e6  Vbase=500e3  OutputType=Complex  PhasorSimulation=off  PSBequivalent=0
  Wind Turbine : Subsystem  AncestorBlock=re_lib/Wind Generation/Wind Turbine  DialogController=POWERSYS.PowerSysDialog  mask(Wind Turbine){Pnom=1.5e6, Pelec_base=1.5e6/0.9, wind_base=12, P_wind_base=0.73, speed_nom=1.2, pitch_angle=0, DisplayTurbChar=off, c1_c6=[0.51763          116          0.4            5           21     0.006795], cp_nom=0.48, lambda_nom=8.1}
      mask prompts: Pnom "Nominal mechanical output power (W):"; Pelec_base "Base power of the electrical generator (VA):"; wind_base "Base wind speed (m/s):"; P_wind_base "Maximum power at base wind speed (pu of nominal mechanical power):"; speed_nom "Base rotational speed (p.u. of base generator speed):"; pitch_angle "Pitch angle beta to display wind-turbine power characteristics (beta >=0)  (deg):"; DisplayTurbChar "Display wind turbine power characteristics"
      mask help:
      | This block implements a variable pitch wind turbine model. The performance coefficient Cp of the turbine is the mechanical output power of the turbine divided by wind power and a function of wind speed, rotational speed, and pitch angle (beta). Cp reaches its maximum value at zero beta. Select the wind-turbine power characteristics display to plot the turbine characteristics at the specified pitch angle.
      |
      | The first input is the generator speed in per unit of the generator base speed. For a synchronous or asynchronous generator, the base speed is the synchronous speed. For a permanent-magnet generator, the base speed is defined as the speed producing nominal voltage at  no load. The second input is the blade pitch angle (beta) in degrees. The third input is the wind speed in m/s.
      |
      | The output is the torque applied to the generator shaft in per unit of the generator ratings.
      |
      | The turbine inertia must be added to the generator inertia.
      mask init: same as HPWnew/Wind Power System 60 KW x 25 = 1.5MW/Wind 60KW, 50HZ, 440V1/Wind Turbine
      mask Help: helpview(psbhelp);
      mask Callback Pnom:
      | ParVisible={'on','on','on','on','on','on','on','off','off','off',};
      | set_param(gcb,'MaskVisibilities',ParVisible);
      | c1_c6=str2num(get_param(gcb,'c1_c6'));
      | c1=c1_c6(1);c2=c1_c6(2);c3=c1_c6(3);c4=c1_c6(4);c5=c1_c6(5);c6=c1_c6(6);
      mask Callback DisplayTurbChar:
      | DisplayTurbChar=get_param(gcb,'DisplayTurbChar');
      | 
      | if strcmp(DisplayTurbChar,'on')
      |     fig_num=figure;
      | 	clf(fig_num);
      | 	[speed_nom,wind_base,P_wind_base,pitch_angle]=getSPSmaskvalues(gcb,{'speed_nom','wind_base','P_wind_base','pitch_angle'});
      | 	[c1_c6,lambda_nom,cp_nom]=getSPSmaskvalues(gcb,{'c1_c6','lambda_nom','cp_nom'});
      | 	c1=c1_c6(1);c2=c1_c6(2);c3=c1_c6(3);c4=c1_c6(4);c5=c1_c6(5);c6=c1_c6(6);
      | 
      | 	%Wind turbine typical characteristic data
      |     %c2=116;c3=0.4;c4=5;c5=21;
      |     %Computation of c1 and c6 for lambda_nom et cpmax
      |     %lambda_nom=8.1;
      |     %cp_max=0.48;
      |     %cp_nom=cp_max;
      | 
      |     %lambda_i_nom=1/(1/lambda_nom-0.035);
      |     %k_nom=-(c2*c5/lambda_i_nom-c4*c5-c2)*exp(-c5/lambda_i_nom)/lambda_nom^2;
      |     %c1=cp_max/((c2/lambda_i_nom-c4)*exp(-c5/lambda_i_nom)+k_nom*lambda_nom);
      |     %c6=k_nom*c1;
      | 
      | 	wr_elec_pu=1e-3:0.01:1.5;;
      |     wr_mec_pu=wr_elec_pu/speed_nom;
      |     wind_max=ceil((1.2/P_wind_base)^(1/3)*wind_base);
      |     wind_min=round(((0.1)/P_wind_base)^(1/3)*wind_base);
      |     wind1=wind_min:(wind_base-wind_min)/5:wind_base;
      |     wind2=wind_base+(wind_base-wind_min)/5:(wind_base-wind_min)/5:wind_max;
      |     wind_pu=[wind1 wind2]/wind_base;
      | 
      |     for k=1:length(wind_pu)
      |         for i=1:length(wr_mec_pu);
      |             lambda_pu=wr_mec_pu(i)/wind_pu(k);
      |             lambda=lambda_pu*lambda_nom;
      |             lambda_i=1/(1/(lambda+0.08*pitch_angle)-0.035/(pitch_angle^3+1));
      |             cp=c1*(c2/lambda_i-c3*pitch_angle-c4)*exp(-c5/lambda_i)+c6*lambda;
      |             cp_pu=cp/cp_nom;
      |             Pwind_pu(k,i)=wind_pu(k)^3*cp_pu*P_wind_base;
      |         end
      |     end
      |     for k=1:length(wind_pu)
      |         plot(wr_elec_pu,Pwind_pu(k,:))
      |         hold on
      |     end
      | 
      |     plot([speed_nom,speed_nom,0],[0,P_wind_base,P_wind_base],'r--')
      |     text(speed_nom+0.01,0+0.05,sprintf('%0.4g pu',speed_nom))
      |     text(0.01,P_wind_base+0.05,sprintf('Max. power at base wind speed (%0.4g m/s) and beta = 0 deg',wind_base))
      |     for i=1:length(wind_pu),
      |         p_max(i)=max(Pwind_pu(i,:));
      |         speed(i)=wr_elec_pu(find(Pwind_pu(i,:)==p_max(i)));
      |         text(speed(i),p_max(i),sprintf('%0.4g m/s',wind_pu(i)*wind_base))
      |     end
      |     plot([0 max(wr_elec_pu)],[0 0],'--')
      | 
      |     xlabel('Turbine speed (pu of nominal generator speed)')
      |     ylabel('Turbine output power (pu of nominal mechanical power)')
      |     title(sprintf('Turbine Power Characteristics (Pitch angle beta = %0.4g deg)',pitch_angle))
      |     axis([0 max(wr_elec_pu) min(Pwind_pu(1,:)) max(P_wind_base+0.1,max(wind_pu)^3*P_wind_base+0.1)])
      |     set_param(gcb,'DisplayTurbChar','off')
      | end
      mask Display: disp('');
  i mach : powerlib/Measurements/Current Measurement  Tag=PoWeRsYsTeMmEaSuReMeNt  PhasorSimulation=off  OutputType=Magnitude  PSBequivalent=0
  iA (A) : Scope
      settings: TickLabels=on  TimeRange=3  YMin=-100  YMax=100  SaveName=is1
  vf : Constant  Value=17.888
  A : PMIOPort  Port=1  Side=Right
  B : PMIOPort  Port=2  Side=Right
  C : PMIOPort  Port=3  Side=Right
  wires:
  Three-Phase V-I Measurement/2 -> Scope/2
  Three-Phase V-I Measurement/1 -> Scope/1
  PA (deg)/1 -> Wind Turbine/2(Pitch angle (deg))
  Wind Speed (m/s)/1 -> Wind Turbine/3(Wind speed (m/s))
  "Gen Speed "/1 -> Wind Turbine/1(Generator speed (pu))
  Wind Turbine/1("Tm ") -> Synchronous Machine 762 V 111.9 kW/1
  vf/1 -> Synchronous Machine 762 V 111.9 kW/2
  i mach/1 -> iA (A)/1
  connections:
  Three-Phase V-I Measurement/LConn3 -- Synchronous Machine 762 V 111.9 kW/RConn3
  Three-Phase V-I Measurement/LConn1 -- Synchronous Machine 762 V 111.9 kW/RConn1
  Three-Phase V-I Measurement/LConn2 -- Synchronous Machine 762 V 111.9 kW/RConn2
  Three-Phase V-I Measurement/RConn1 -- i mach/LConn1
  Ground (output)/LConn1 -- Network 440Vrms LN - 10 MVA/LConn1
  i mach/RConn1 -- Three-Phase Series RLC Load/LConn1 -- Load Flow Bus/LConn1 -- Network 440Vrms LN - 10 MVA/RConn1 -- A/RConn1
  Three-Phase Series RLC Load/LConn3 -- Three-Phase V-I Measurement/RConn3 -- Network 440Vrms LN - 10 MVA/RConn3 -- C/RConn1
  Network 440Vrms LN - 10 MVA/RConn2 -- Three-Phase V-I Measurement/RConn2 -- Three-Phase Series RLC Load/LConn2 -- B/RConn1

== system HPWnew/Wind Power System 60 KW x 25 = 1.5MW/Wind 60KW, 50HZ, 440V22 ==
  "Gen Speed " : Inport
  PA (deg) : Inport  Port=2
  Wind Speed (m/s) : Inport  Port=3
  Ground (output) : powerlib/Elements/Ground  LConnTagsString=a
  Load Flow Bus : powerlib/Measurements/Load Flow Bus  LConnTagsString=a  ID=B1  Vbase=762.1  Vref=1  Vangle=0  VLF=1  angleLF=-0.3472
      settings: AttributesFormatString=%<ID>\n%<Vbase>V\n%<VLF>pu\n%<angleLF>deg.
  Network 440Vrms LN - 10 MVA : powerlib/Electrical Sources/Three-Phase Source  Voltage=(762.1)*1  PhaseAngle=0  Frequency=60  InternalConnection=Yn  SpecifyImpedance=off  Resistance=762^2/10e6/10  Inductance=762^2/10e6/(2*pi*60)  ShortCircuitLevel=100e6  BaseVoltage=25e3  XRratio=7  BusType=swing  Pref=0  Qref=0  Qmin=-Inf  Qmax=Inf
  Scope : Scope  NumInputPorts=2
      settings: TimeRange=0.05586047612700701  YMin=-800~-200  YMax=800~200
  Synchronous Machine 762 V 111.9 kW : powerlib/Machines/Synchronous Machine SI Fundamental  PresetModel=05: 50Hz 400V 60kVA 1500RPM  MechanicalLoad=Mechanical power Pm  ShowDetailedParameters=on  RotorType=Salient-pole  Units=SI fundamental parameters  MeasurementBus=off  NominalParameters=[6e+04 400 50]  Stator=[0.101 0.0006791 0.01833 0.007979]  Field=[0.05664 0.001459]  Dampers2=[ 1 2 3 4 5 6 ]  Dampers1=[0.3901 0.002619 0.1534 0.0004483]  Mechanical=[0.5 0.05 2]  PolePairs=2  InitialConditions=[0 -111.483 53.977 53.977 53.977 -173.297 -293.297 -53.2967 17.8876]  SetSaturation=off  Saturation=[46.376,51.647,61.167,66.773,72.147,78.393,86.24,95.347,105.58;644,708.2,816.2,870.87,917.13,962.47,1012,1059.3,1104.5]  DisplayVfd=off  LoadFlowParameters=[1 -50000 0 0 0]  TsPowergui=0  TsBlock=-1  IterativeModel=Forward Euler  BusType=PV  Pref=-50000  Qref=0  Qmin=-Inf  Qmax=Inf  PLF=0  QLF=0
      settings: AttributesFormatString=\n
  Three-Phase Series RLC Load : powerlib/Elements/Three-Phase Series RLC Load  LConnTagsString=A|B|C  Configuration=Y (grounded)  NominalVoltage=440  NominalFrequency=50  ActivePower=10e3  InductivePower=0  CapacitivePower=0  Measurements=None  LoadType=constant Z
  Three-Phase V-I Measurement : powerlib/Measurements/Three-Phase V-I Measurement  VoltageMeasurement=phase-to-ground  SetLabelV=off  LabelV=Vabc  Vpu=off  VpuLL=off  CurrentMeasurement=yes  SetLabelI=off  LabelI=Iabc  Ipu=off  Pbase=100e6  Vbase=500e3  OutputType=Complex  PhasorSimulation=off  PSBequivalent=0
  Wind Turbine : Subsystem  AncestorBlock=re_lib/Wind Generation/Wind Turbine  DialogController=POWERSYS.PowerSysDialog  mask(Wind Turbine){Pnom=1.5e6, Pelec_base=1.5e6/0.9, wind_base=12, P_wind_base=0.73, speed_nom=1.2, pitch_angle=0, DisplayTurbChar=off, c1_c6=[0.51763          116          0.4            5           21     0.006795], cp_nom=0.48, lambda_nom=8.1}
      mask prompts: Pnom "Nominal mechanical output power (W):"; Pelec_base "Base power of the electrical generator (VA):"; wind_base "Base wind speed (m/s):"; P_wind_base "Maximum power at base wind speed (pu of nominal mechanical power):"; speed_nom "Base rotational speed (p.u. of base generator speed):"; pitch_angle "Pitch angle beta to display wind-turbine power characteristics (beta >=0)  (deg):"; DisplayTurbChar "Display wind turbine power characteristics"
      mask help:
      | This block implements a variable pitch wind turbine model. The performance coefficient Cp of the turbine is the mechanical output power of the turbine divided by wind power and a function of wind speed, rotational speed, and pitch angle (beta). Cp reaches its maximum value at zero beta. Select the wind-turbine power characteristics display to plot the turbine characteristics at the specified pitch angle.
      |
      | The first input is the generator speed in per unit of the generator base speed. For a synchronous or asynchronous generator, the base speed is the synchronous speed. For a permanent-magnet generator, the base speed is defined as the speed producing nominal voltage at  no load. The second input is the blade pitch angle (beta) in degrees. The third input is the wind speed in m/s.
      |
      | The output is the torque applied to the generator shaft in per unit of the generator ratings.
      |
      | The turbine inertia must be added to the generator inertia.
      mask init: same as HPWnew/Wind Power System 60 KW x 25 = 1.5MW/Wind 60KW, 50HZ, 440V1/Wind Turbine
      mask Help: helpview(psbhelp);
      mask Callback Pnom:
      | ParVisible={'on','on','on','on','on','on','on','off','off','off',};
      | set_param(gcb,'MaskVisibilities',ParVisible);
      | c1_c6=str2num(get_param(gcb,'c1_c6'));
      | c1=c1_c6(1);c2=c1_c6(2);c3=c1_c6(3);c4=c1_c6(4);c5=c1_c6(5);c6=c1_c6(6);
      mask Callback DisplayTurbChar:
      | DisplayTurbChar=get_param(gcb,'DisplayTurbChar');
      | 
      | if strcmp(DisplayTurbChar,'on')
      |     fig_num=figure;
      | 	clf(fig_num);
      | 	[speed_nom,wind_base,P_wind_base,pitch_angle]=getSPSmaskvalues(gcb,{'speed_nom','wind_base','P_wind_base','pitch_angle'});
      | 	[c1_c6,lambda_nom,cp_nom]=getSPSmaskvalues(gcb,{'c1_c6','lambda_nom','cp_nom'});
      | 	c1=c1_c6(1);c2=c1_c6(2);c3=c1_c6(3);c4=c1_c6(4);c5=c1_c6(5);c6=c1_c6(6);
      | 
      | 	%Wind turbine typical characteristic data
      |     %c2=116;c3=0.4;c4=5;c5=21;
      |     %Computation of c1 and c6 for lambda_nom et cpmax
      |     %lambda_nom=8.1;
      |     %cp_max=0.48;
      |     %cp_nom=cp_max;
      | 
      |     %lambda_i_nom=1/(1/lambda_nom-0.035);
      |     %k_nom=-(c2*c5/lambda_i_nom-c4*c5-c2)*exp(-c5/lambda_i_nom)/lambda_nom^2;
      |     %c1=cp_max/((c2/lambda_i_nom-c4)*exp(-c5/lambda_i_nom)+k_nom*lambda_nom);
      |     %c6=k_nom*c1;
      | 
      | 	wr_elec_pu=1e-3:0.01:1.5;;
      |     wr_mec_pu=wr_elec_pu/speed_nom;
      |     wind_max=ceil((1.2/P_wind_base)^(1/3)*wind_base);
      |     wind_min=round(((0.1)/P_wind_base)^(1/3)*wind_base);
      |     wind1=wind_min:(wind_base-wind_min)/5:wind_base;
      |     wind2=wind_base+(wind_base-wind_min)/5:(wind_base-wind_min)/5:wind_max;
      |     wind_pu=[wind1 wind2]/wind_base;
      | 
      |     for k=1:length(wind_pu)
      |         for i=1:length(wr_mec_pu);
      |             lambda_pu=wr_mec_pu(i)/wind_pu(k);
      |             lambda=lambda_pu*lambda_nom;
      |             lambda_i=1/(1/(lambda+0.08*pitch_angle)-0.035/(pitch_angle^3+1));
      |             cp=c1*(c2/lambda_i-c3*pitch_angle-c4)*exp(-c5/lambda_i)+c6*lambda;
      |             cp_pu=cp/cp_nom;
      |             Pwind_pu(k,i)=wind_pu(k)^3*cp_pu*P_wind_base;
      |         end
      |     end
      |     for k=1:length(wind_pu)
      |         plot(wr_elec_pu,Pwind_pu(k,:))
      |         hold on
      |     end
      | 
      |     plot([speed_nom,speed_nom,0],[0,P_wind_base,P_wind_base],'r--')
      |     text(speed_nom+0.01,0+0.05,sprintf('%0.4g pu',speed_nom))
      |     text(0.01,P_wind_base+0.05,sprintf('Max. power at base wind speed (%0.4g m/s) and beta = 0 deg',wind_base))
      |     for i=1:length(wind_pu),
      |         p_max(i)=max(Pwind_pu(i,:));
      |         speed(i)=wr_elec_pu(find(Pwind_pu(i,:)==p_max(i)));
      |         text(speed(i),p_max(i),sprintf('%0.4g m/s',wind_pu(i)*wind_base))
      |     end
      |     plot([0 max(wr_elec_pu)],[0 0],'--')
      | 
      |     xlabel('Turbine speed (pu of nominal generator speed)')
      |     ylabel('Turbine output power (pu of nominal mechanical power)')
      |     title(sprintf('Turbine Power Characteristics (Pitch angle beta = %0.4g deg)',pitch_angle))
      |     axis([0 max(wr_elec_pu) min(Pwind_pu(1,:)) max(P_wind_base+0.1,max(wind_pu)^3*P_wind_base+0.1)])
      |     set_param(gcb,'DisplayTurbChar','off')
      | end
      mask Display: disp('');
  i mach : powerlib/Measurements/Current Measurement  Tag=PoWeRsYsTeMmEaSuReMeNt  PhasorSimulation=off  OutputType=Magnitude  PSBequivalent=0
  iA (A) : Scope
      settings: TickLabels=on  TimeRange=3  YMin=-100  YMax=100  SaveName=is1
  vf : Constant  Value=17.888
  A : PMIOPort  Port=1  Side=Right
  B : PMIOPort  Port=2  Side=Right
  C : PMIOPort  Port=3  Side=Right
  wires:
  i mach/1 -> iA (A)/1
  vf/1 -> Synchronous Machine 762 V 111.9 kW/2
  Wind Turbine/1("Tm ") -> Synchronous Machine 762 V 111.9 kW/1
  "Gen Speed "/1 -> Wind Turbine/1(Generator speed (pu))
  Wind Speed (m/s)/1 -> Wind Turbine/3(Wind speed (m/s))
  PA (deg)/1 -> Wind Turbine/2(Pitch angle (deg))
  Three-Phase V-I Measurement/1 -> Scope/1
  Three-Phase V-I Measurement/2 -> Scope/2
  connections:
  B/RConn1 -- Three-Phase Series RLC Load/LConn2 -- Three-Phase V-I Measurement/RConn2 -- Network 440Vrms LN - 10 MVA/RConn2
  C/RConn1 -- Network 440Vrms LN - 10 MVA/RConn3 -- Three-Phase V-I Measurement/RConn3 -- Three-Phase Series RLC Load/LConn3
  A/RConn1 -- Network 440Vrms LN - 10 MVA/RConn1 -- Load Flow Bus/LConn1 -- Three-Phase Series RLC Load/LConn1 -- i mach/RConn1
  Ground (output)/LConn1 -- Network 440Vrms LN - 10 MVA/LConn1
  Three-Phase V-I Measurement/RConn1 -- i mach/LConn1
  Three-Phase V-I Measurement/LConn2 -- Synchronous Machine 762 V 111.9 kW/RConn2
  Three-Phase V-I Measurement/LConn1 -- Synchronous Machine 762 V 111.9 kW/RConn1
  Three-Phase V-I Measurement/LConn3 -- Synchronous Machine 762 V 111.9 kW/RConn3
